simulink model "MotMappedP2"  (R2022a)
settings: Solver=VariableStepAuto  StartTime=0.0  StopTime=inf  RelTol=1e-3  EnableMultiTasking=on
model workspace (MAT data in the model file):
  EV_current = Simulink.Parameter
  EV_current.Value = 200
  EV_current.DataType = 'double'
  EV_current.Complexity = 'real'
  EV_current.Dimensions = [1 1]
  EV_motion = Simulink.Parameter
  EV_motion.Value = [20 4 0.8]
  EV_motion.DataType = 'double'
  EV_motion.Complexity = 'real'
  EV_motion.Dimensions = [1 3]
  EV_sf = Simulink.Parameter
  EV_sf.Value = 2000
  EV_sf.DataType = 'double'
  EV_sf.Complexity = 'real'
  EV_sf.Dimensions = [1 1]
  Fs = Simulink.Parameter
  Fs.Value = 0
  Fs.DataType = 'double'
  Fs.Complexity = 'real'
  Fs.Dimensions = [1 1]
  Fv = Simulink.Parameter
  Fv.Value = 0.0025
  Fv.DataType = 'double'
  Fv.Complexity = 'real'
  Fv.Dimensions = [1 1]
  Jcomp = Simulink.Parameter
  Jcomp.Value = 0.0227
  Jcomp.DataType = 'double'
  Jcomp.Complexity = 'real'
  Jcomp.Dimensions = [1 1]
  Ki = Simulink.Parameter
  Ki.Value = 251.3274
  Ki.DataType = 'double'
  Ki.Complexity = 'real'
  Ki.Dimensions = [1 1]
  Kisa = Simulink.Parameter
  Kisa.Value = 346.6583
  Kisa.DataType = 'double'
  Kisa.Complexity = 'real'
  Kisa.Dimensions = [1 1]
  Kp_d = Simulink.Parameter
  Kp_d.Value = 0.47149
  Kp_d.DataType = 'double'
  Kp_d.Complexity = 'real'
  Kp_d.Dimensions = [1 1]
  Kp_q = Simulink.Parameter
  Kp_q.Value = 0.52125
  Kp_q.DataType = 'double'
  Kp_q.Complexity = 'real'
  Kp_q.Dimensions = [1 1]
  Ksa = Simulink.Parameter
  Ksa.Value = 85.4316
  Ksa.DataType = 'double'
  Ksa.Complexity = 'real'
  Ksa.Dimensions = [1 1]
  Ksf = Simulink.Parameter
  Ksf.Value = 1996.2651
  Ksf.DataType = 'double'
  Ksf.Complexity = 'real'
  Ksf.Dimensions = [1 1]
  Ld = Simulink.Parameter
  Ld.Value = 0.0003752
  Ld.DataType = 'double'
  Ld.Complexity = 'real'
  Ld.Dimensions = [1 1]
  Ldq = Simulink.Parameter
  Ldq.Value = [0.0003752 0.0004148]
  Ldq.DataType = 'double'
  Ldq.Complexity = 'real'
  Ldq.Dimensions = [1 2]
  Lq = Simulink.Parameter
  Lq.Value = 0.0004148
  Lq.DataType = 'double'
  Lq.Complexity = 'real'
  Lq.Dimensions = [1 1]
  Mechanical = Simulink.Parameter
  Mechanical.Value = [0.0227 0.0025 0]
  Mechanical.DataType = 'double'
  Mechanical.Complexity = 'real'
  Mechanical.Dimensions = [1 3]
  P = Simulink.Parameter
  P.Value = 4
  P.DataType = 'double'
  P.Complexity = 'real'
  P.Dimensions = [1 1]
  PolePairs = Simulink.Parameter
  PolePairs.Value = 4
  PolePairs.DataType = 'double'
  PolePairs.Complexity = 'real'
  PolePairs.Dimensions = [1 1]
  Rs = Simulink.Parameter
  Rs.Value = 0.2
  Rs.DataType = 'double'
  Rs.Complexity = 'real'
  Rs.Dimensions = [1 1]
  T_eff_bp = Simulink.Parameter
  T_eff_bp.Value = [0 20 40 60 80 100 120 140 160 180 200]
  T_eff_bp.DataType = 'double'
  T_eff_bp.Complexity = 'real'
  T_eff_bp.Dimensions = [1 11]
  T_max = Simulink.Parameter
  T_max.Value = 120
  T_max.DataType = 'double'
  T_max.Complexity = 'real'
  T_max.Dimensions = [1 1]
  T_mtpa = Simulink.Parameter
  T_mtpa.Value = [0 13.3131834767 26.6278836885 39.9456159322 53.2678926341 66.5962219318 79.9321062746 93.277041051 106.632513247 120.000000141]
  T_mtpa.DataType = 'double'
  T_mtpa.Complexity = 'real'
  T_mtpa.Dimensions = [1 10]
  Tc = Simulink.Parameter
  Tc.Value = 0.02
  Tc.DataType = 'double'
  Tc.Complexity = 'real'
  Tc.Dimensions = [1 1]
  Temp_eff_bp = Simulink.Parameter
  Temp_eff_bp.Value = [233.15 293.15 373.15]
  Temp_eff_bp.DataType = 'double'
  Temp_eff_bp.Complexity = 'real'
  Temp_eff_bp.Dimensions = [1 3]
  ba = Simulink.Parameter
  ba.Value = 3.4029
  ba.DataType = 'double'
  ba.Complexity = 'real'
  ba.Dimensions = [1 1]
  efficiency_table = Simulink.Parameter
  efficiency_table.Value = [52  78  80  82  82  80  78  78  76  74  70; 52  78  80  82  82  80  78  78  76  74  70; 52  78  84  86  86  86  86  84  84  82  82; 52  80  86  86  88  88  88  86  86  84  84; 52  80  86  88  88  88  88  88  86  86  86; 52  80  86  88  90  90  90  90  88  88  88; 52  82  88  90  91  91  92  92  92  91  91; 52  82  88  91  91  92  93  93  93  93  93; 52  84  90  92  92  93  93  93  93  93  93; 62  86  91  93  93  93  93  93  93  93  93; 66  86  91  93  93  93  93  93  93  93  93; 70  86  92  93  93  93  93  93  93  93  93; 70  86  92  93  93  93  93  93  93  93  93; 72  86  91  93  93  93  93  93  93  93  93]
  efficiency_table.DataType = 'double'
  efficiency_table.Complexity = 'real'
  efficiency_table.Dimensions = [14 11]
  efficiency_table_3d = Simulink.Parameter
  efficiency_table_3d.Value = reshape([92 92 92 92 92 92 92 92 92 92 92 92 92 92 92 92 92 92 92 92 92 92 92 92 92 92 92 92 92 92 92 92 92 92 92 92 92 92 92 92 92 92 92 92 92 92 92 92 92 92 92 92 92 92 92 92 92 92 92 92 92 92 92 92 92 92 92 92 92 92 92 92 92 92 92 92 92 92 92 92 92 92 92 92 92 92 92 92 92 92 92 92 92 92 92 92 92 92 92 92 92 92 92 92 92 92 92 92 92 92 92 92 92 92 92 92 92 92 92 92 92 92 92 92 92 92 92 92 92 92 92 92 92 92 92 92 92 92 92 92 92 92 92 92 92 92 92 92 92 92 92 92 92 92 95 95 95 95 95 95 95 95 95 95 95 95 95 95 95 95 95 95 95 95 95 95 95 95 95 95 95 95 95 95 95 95 95 95 95 95 95 95 95 95 95 95 95 95 95 95 95 95 95 95 95 95 95 95 95 95 95 95 95 95 95 95 95 95 95 95 95 95 95 95 95 95 95 95 95 95 95 95 95 95 95 95 95 95 95 95 95 95 95 95 95 95 95 95 95 95 95 95 95 95 95 95 95 95 95 95 95 95 95 95 95 95 95 95 95 95 95 95 95 95 95 95 95 95 95 95 95 95 95 95 95 95 95 95 95 95 95 95 95 95 95 95 95 95 95 95 95 95 95 95 95 95 95 95 93 93 93 93 93 93 93 93 93 93 93 93 93 93 93 93 93 93 93 93 93 93 93 93 93 93 93 93 93 93 93 93 93 93 93 93 93 93 93 93 93 93 93 93 93 93 93 93 93 93 93 93 93 93 93 93 93 93 93 93 93 93 93 93 93 93 93 93 93 93 93 93 93 93 93 93 93 93 93 93 93 93 93 93 93 93 93 93 93 93 93 93 93 93 93 93 93 93 93 93 93 93 93 93 93 93 93 93 93 93 93 93 93 93 93 93 93 93 93 93 93 93 93 93 93 93 93 93 93 93 93 93 93 93 93 93 93 93 93 93 93 93 93 93 93 93 93 93 93 93 93 93 93 93], [14 11 3])
  efficiency_table_3d.DataType = 'double'
  efficiency_table_3d.Complexity = 'real'
  efficiency_table_3d.Dimensions = [14 11 3]
  id_mtpa = Simulink.Parameter
  id_mtpa.Value = [0 -0.114523352646 -0.457989076459 -1.03008464374 -1.83029075221 -2.85788367342 -4.11193850568 -5.59133329791 -7.29475400168 -9.22070020138]
  id_mtpa.DataType = 'double'
  id_mtpa.Complexity = 'real'
  id_mtpa.Dimensions = [1 10]
  idq0 = Simulink.Parameter
  idq0.Value = [0 0]
  idq0.DataType = 'double'
  idq0.Complexity = 'real'
  idq0.Dimensions = [1 2]
  idq_limits = Simulink.Parameter
  idq_limits.Value = [-9.220699542 166.993501392 167.247872355]
  idq_limits.DataType = 'double'
  idq_limits.Complexity = 'real'
  idq_limits.Dimensions = [1 3]
  iq_mtpa = Simulink.Parameter
  iq_mtpa.Value = [0 18.5827440345 37.1633719111 55.7397734896 74.3098506185 92.871523015 111.422734008 129.961456105 148.485696337 166.993501356]
  iq_mtpa.DataType = 'double'
  iq_mtpa.Complexity = 'real'
  iq_mtpa.Dimensions = [1 10]
  lambda_pm = Simulink.Parameter
  lambda_pm.Value = 0.1194
  lambda_pm.DataType = 'double'
  lambda_pm.Complexity = 'real'
  lambda_pm.Dimensions = [1 1]
  losses_table = Simulink.Parameter
  losses_table.Value = [0 0 0 0 0 0 0 0 0 0 0 0 ... (154 elements, 14x11)]
  losses_table.DataType = 'double'
  losses_table.Complexity = 'real'
  losses_table.Dimensions = [14 11]
  losses_table_3d = Simulink.Parameter
  losses_table_3d.Value = reshape([2 2 2 2 2 2 2 2 2 2 2 2 2 2 2 2 2 2 2 2 2 2 2 2 2 2 2 2 2 2 2 2 2 2 2 2 2 2 2 2 2 2 2 2 2 2 2 2 2 2 2 2 2 2 2 2 2 2 2 2 2 2 2 2 2 2 2 2 2 2 2 2 2 2 2 2 2 2 2 2 2 2 2 2 2 2 2 2 2 2 2 2 2 2 2 2 2 2 2 2 2 2 2 2 2 2 2 2 2 2 2 2 2 2 2 2 2 2 2 2 2 2 2 2 2 2 2 2 2 2 2 2 2 2 2 2 2 2 2 2 2 2 2 2 2 2 2 2 2 2 2 2 2 2 1.5 1.5 1.5 1.5 1.5 1.5 1.5 1.5 1.5 1.5 1.5 1.5 1.5 1.5 1.5 1.5 1.5 1.5 1.5 1.5 1.5 1.5 1.5 1.5 1.5 1.5 1.5 1.5 1.5 1.5 1.5 1.5 1.5 1.5 1.5 1.5 1.5 1.5 1.5 1.5 1.5 1.5 1.5 1.5 1.5 1.5 1.5 1.5 1.5 1.5 1.5 1.5 1.5 1.5 1.5 1.5 1.5 1.5 1.5 1.5 1.5 1.5 1.5 1.5 1.5 1.5 1.5 1.5 1.5 1.5 1.5 1.5 1.5 1.5 1.5 1.5 1.5 1.5 1.5 1.5 1.5 1.5 1.5 1.5 1.5 1.5 1.5 1.5 1.5 1.5 1.5 1.5 1.5 1.5 1.5 1.5 1.5 1.5 1.5 1.5 1.5 1.5 1.5 1.5 1.5 1.5 1.5 1.5 1.5 1.5 1.5 1.5 1.5 1.5 1.5 1.5 1.5 1.5 1.5 1.5 1.5 1.5 1.5 1.5 1.5 1.5 1.5 1.5 1.5 1.5 1.5 1.5 1.5 1.5 1.5 1.5 1.5 1.5 1.5 1.5 1.5 1.5 1.5 1.5 1.5 1.5 1.5 1.5 1.5 1.5 1.5 1.5 1.5 1.5 1.9 1.9 1.9 1.9 1.9 1.9 1.9 1.9 1.9 1.9 1.9 1.9 1.9 1.9 1.9 1.9 1.9 1.9 1.9 1.9 1.9 1.9 1.9 1.9 1.9 1.9 1.9 1.9 1.9 1.9 1.9 1.9 1.9 1.9 1.9 1.9 1.9 1.9 1.9 1.9 1.9 1.9 1.9 1.9 1.9 1.9 1.9 1.9 1.9 1.9 1.9 1.9 1.9 1.9 1.9 1.9 1.9 1.9 1.9 1.9 1.9 1.9 1.9 1.9 1.9 1.9 1.9 1.9 1.9 1.9 1.9 1.9 1.9 1.9 1.9 1.9 1.9 1.9 1.9 1.9 1.9 1.9 1.9 1.9 1.9 1.9 1.9 1.9 1.9 1.9 1.9 1.9 1.9 1.9 1.9 1.9 1.9 1.9 1.9 1.9 1.9 1.9 1.9 1.9 1.9 1.9 1.9 1.9 1.9 1.9 1.9 1.9 1.9 1.9 1.9 1.9 1.9 1.9 1.9 1.9 1.9 1.9 1.9 1.9 1.9 1.9 1.9 1.9 1.9 1.9 1.9 1.9 1.9 1.9 1.9 1.9 1.9 1.9 1.9 1.9 1.9 1.9 1.9 1.9 1.9 1.9 1.9 1.9 1.9 1.9 1.9 1.9 1.9 1.9], [14 11 3])
  losses_table_3d.DataType = 'double'
  losses_table_3d.Complexity = 'real'
  losses_table_3d.Dimensions = [14 11 3]
  mechanical = Simulink.Parameter
  mechanical.Value = [0.0227 0.0025 0]
  mechanical.DataType = 'double'
  mechanical.Complexity = 'real'
  mechanical.Dimensions = [1 3]
  omega_init = Simulink.Parameter
  omega_init.Value = 0
  omega_init.DataType = 'double'
  omega_init.Complexity = 'real'
  omega_init.Dimensions = [1 1]
  power_max = Simulink.Parameter
  power_max.Value = 30000
  power_max.DataType = 'double'
  power_max.Complexity = 'real'
  power_max.Dimensions = [1 1]
  theta_init = Simulink.Parameter
  theta_init.Value = 0
  theta_init.DataType = 'double'
  theta_init.Complexity = 'real'
  theta_init.Dimensions = [1 1]
  torque_max = Simulink.Parameter
  torque_max.Value = 200
  torque_max.DataType = 'double'
  torque_max.Complexity = 'real'
  torque_max.Dimensions = [1 1]
  w_eff_bp = Simulink.Parameter
  w_eff_bp.Value = [0 52.3598775598 104.71975512 149.999649207 157.079632679 209.439510239 261.799387799 314.159265359 366.519142919 418.879020479 471.238898038 523.598775598 575.958653158 628.318530718]
  w_eff_bp.DataType = 'double'
  w_eff_bp.Complexity = 'real'
  w_eff_bp.Dimensions = [1 14]
libraries: autolibmappedmotor x1
settings Model: DataDictionary=MotMappedP2.sldd  ModifiedByFormat=The MathWorks, Inc.  PauseTimes=10  Creator=The MathWorks, Inc.  LastModifiedBy=The MathWorks, Inc.
settings SolverCC: AlgebraicLoopSolver=TrustRegion  AutoInsertRateTranBlk=on  DecoupledContinuousIntegration=on  MaxZcPerStep=1
settings DataIOCC: DSMLogging=off  ReturnWorkspaceOutputs=off
settings DebuggingCC: UnconnectedInputMsg=warning  UnconnectedOutputMsg=warning  UnconnectedLineMsg=warning  PregeneratedLibrarySubsystemCodeDiagnostic=none  SFMachineParentedDataDiag=warning  ArithmeticOperatorsInVariantConditions=warning
settings ModelReferenceCC: PropagateSignalLabelsOutOfModel=off
settings SFSimCC: SimUseLocalCustomCode=off  CustomCodeUndefinedFunction=UseInterfaceOnly
settings RTWCC: RTWUseLocalCustomCode=off  DLArmComputeVersion=19.05
settings CodeAppCC: StateflowObjectComments=on
settings GRTTargetCC: TargetLangStandard=C89/C90 (ANSI)
settings ConfigComp: CovMetricSettings=dsw  CovSaveCumulativeToWorkspaceVar=on  CovSaveSingleToWorkspaceVar=on  CovExternalEMLEnable=off
settings SimscapeCC: SimscapeNormalizeSystem=off

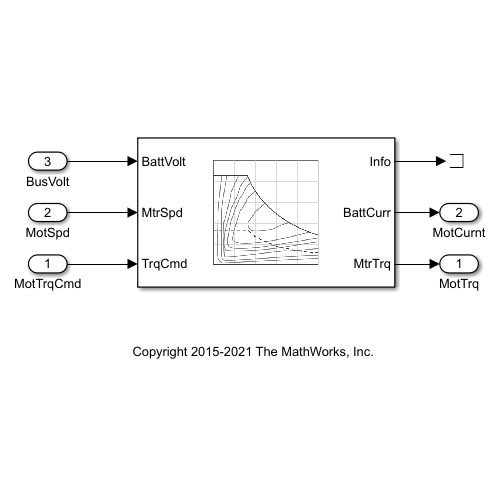
[thumbnail: Simulink's stored preview of the top-level diagram]
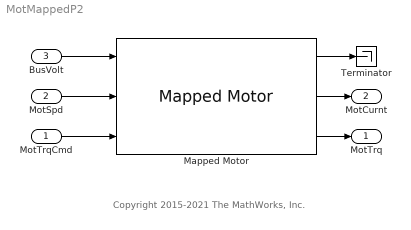
== system MotMappedP2 ==
  note: Copyright 2015-2021 The MathWorks, Inc.
  MotTrqCmd : Inport
  MotSpd : Inport  Port=2
  BusVolt : Inport  Port=3
  Mapped Motor : autolibmappedmotor/Mapped Motor  port_config=Speed  param_by=Maximum torque and power  w_t=[ 0 375 750 800 ]  T_t=[0.09 0.08 0.07 0]  torque_max=torque_max  power_max=power_max  Tc=Tc  param_loss=Tabulated efficiency data  eff=100  w_eff=375  T_eff=0.08  Piron=0  Pbase=0  w_eff_bp=w_eff_bp  T_eff_bp=T_eff_bp  Temp_eff_bp=Temp_eff_bp  losses_table=losses_table  losses_table_3d=losses_table_3d  efficiency_table=efficiency_table  efficiency_table_3d=efficiency_table_3d  J=5e-6  b=1e-5  omega_o=0  T_t_extended=[0 0.07 0.08 0.09 0.08 0.07 0]  w_t_extended=[-800 -750 -375 0 375 750 800]  KLossIron=0  KLossCopper=0  x_w_eff_vec=[-628.318530717959 -575.958653158129 -523.598775598299 -471.238898038469 -418.879020478639 -366.519142918809 -314.159265358979 -261.799387799149 -209.43951023932 -157.07963267949 -149.999649206931 -104.71975511966 -52.3598775598299 0 52.3598775598299 104.71975511966 149.999649206931 157.07963267949 209.43951023932 261.799387799149 314.159265358979 366.519142918809 418.879020478639 471.238898038469 523.598775598299 575.958653158129 628.318530717959]  x_T_eff_vec=[-200 -180 -160 -140 -120 -100 -80 -60 -40 -20 0 20 40 60 80 100 120 140 160 180 200]  x_tmp_eff_vec=[233.15 293.15 373.15]  x_losses_mat=[9458.558526937 8512.7026742433 7566.8468215496 6620.9909688559 5675.1351161622 4729.2792634685 3783.4234107748 2837.5675580811 2485.6557259172 2045.68823954684 0 1759.29188601028 2261.94671058465 2638.93782901542 3518.58377202057 4398.22971502571 5277.87565803085 6157.52160103599 7037.16754404113 7916.81348704627 8796.45943005141;8670.34531635892 7803.31078472303 6936.27625308713 6069.24172145124 5202.20718981535 4335.17265817946 3468.13812654357 2601.10359490768 2003.3344457674 1875.21421958461 0 1612.68422884276 1843.06769010601 2419.02634326414 3225.36845768552 4031.7105721069 4838.05268652828 5644.39480094966 6450.73691537104 7257.07902979242 8063.4211442138;7882.13210578084 7093.91889520275 6305.70568462467 5517.49247404659 4729.2792634685 3941.06605289042 3152.85284231233 2364.63963173425 1821.21313251582 1704.74019962237 0 1466.07657167524 1675.51608191456 2199.11485751285 2932.15314335047 3665.19142918809 4398.22971502571 5131.26800086333 5864.30628670094 6597.34457253856 7330.38285837618;7093.91889520275 6384.52700568248 5675.1351161622 4965.74322664193 4256.35133712165 3546.95944760138 2837.5675580811 2128.17566856083 1864.2417944379 1534.26617966013 0 1319.46891450771 1696.46003293849 1979.20337176157 2638.93782901542 3298.67228626928 3958.40674352314 4618.14120077699 5277.87565803085 5937.61011528471 6597.34457253856;6305.70568462467 5675.1351161622 5044.56454769974 4413.99397923727 3783.4234107748 3152.85284231233 2522.28227384987 1891.7117053874 1657.10381727813 1363.7921596979 0 1172.86125734019 1507.9644737231 1759.29188601028 2345.72251468038 2932.15314335047 3518.58377202057 4105.01440069066 4691.44502936075 5277.87565803085 5864.30628670094;5517.49247404658 4965.74322664193 4413.99397923727 3862.24473183261 3310.49548442795 2758.74623702329 2549.69838552215 1912.27378914161 1628.97396852804 1396.26340159546 0 1172.86125734019 1466.07657167524 1759.29188601028 2345.72251468038 2565.63400043166 3078.76080051799 3591.88760060433 4105.01440069066 4618.14120077699 5131.26800086332;4729.2792634685 4256.35133712165 3783.4234107748 3310.49548442795 2837.5675580811 2731.81969877373 2485.6557259172 1864.2417944379 1713.59599286716 1379.23579913698 0 1130.97335529233 1507.9644737231 1696.46003293849 2261.94671058465 2513.27412287183 2638.93782901542 3078.760800518 3518.58377202057 3958.40674352314 4398.22971502571;5178.44942899416 4660.60448609474 3642.42626503164 3187.12298190269 2731.81969877373 2589.22471449708 2071.37977159766 1745.32925199433 1427.99666072263 1149.36316594749 0 942.477796076938 1256.63706143592 1570.7963267949 1884.95559215388 2356.19449019234 2513.27412287183 2932.15314335047 3351.03216382911 4241.15008234622 4712.38898038469;5711.98664289054 5140.78797860148 4569.58931431243 3257.94793705608 2792.52680319093 2327.10566932577 1861.68453546062 1713.59599286716 1363.7921596979 1047.1975511966 0 837.758040957278 1172.86125734019 1507.9644737231 1675.51608191456 2094.39510239319 2513.27412287183 2932.15314335047 4021.23859659494 4523.8934211693 5026.54824574367;5114.22059886711 4602.7985389804 4091.37647909369 2998.79298751753 2570.39398930074 2141.99499108395 1713.59599286716 1285.19699465037 1022.84411977342 785.398163397448 0 628.318530717959 879.645943005142 1130.97335529233 1507.9644737231 1884.95559215388 2261.94671058465 2638.93782901543 3518.58377202057 3958.40674352314 4398.22971502571;5714.27235074022 5142.8451156662 3906.96760725029 3418.596656344 2454.53971429523 2045.44976191269 1636.35980953016 1465.11285271886 976.741901812573 749.998246034654 0 599.998596827723 839.998035558812 1259.99705333822 1439.99663238654 1799.99579048317 2159.9949485798 2939.99312445584 3359.99214223525 4319.98989715961 4799.98877462179;4597.45266378994 4137.70739741095 3191.45920364677 2792.52680319093 2045.68823954684 1704.74019962237 1363.7921596979 1022.84411977342 797.864800911693 590.726823751927 0 460.766922526503 670.206432765823 879.645943005142 1172.86125734019 1466.07657167524 1759.29188601028 ...(+4852 chars)]  x_losses_mat_3d=cat(3,[2 2 2 2 2 2 2 2 2 2 2 2 2 2 2 2 2 2 2 2 2;2 2 2 2 2 2 2 2 2 2 2 2 2 2 2 2 2 2 2 2 2;2 2 2 2 2 2 2 2 2 2 2 2 2 2 2 2 2 2 2 2 2;2 2 2 2 2 2 2 2 2 2 2 2 2 2 2 2 2 2 2 2 2;2 2 2 2 2 2 2 2 2 2 2 2 2 2 2 2 2 2 2 2 2;2 2 2 2 2 2 2 2 2 2 2 2 2 2 2 2 2 2 2 2 2;2 2 2 2 2 2 2 2 2 2 2 2 2 2 2 2 2 2 2 2 2;2 2 2 2 2 2 2 2 2 2 2 2 2 2 2 2 2 2 2 2 2;2 2 2 2 2 2 2 2 2 2 2 2 2 2 2 2 2 2 2 2 2;2 2 2 2 2 2 2 2 2 2 2 2 2 2 2 2 2 2 2 2 2;2 2 2 2 2 2 2 2 2 2 2 2 2 2 2 2 2 2 2 2 2;2 2 2 2 2 2 2 2 2 2 2 2 2 2 2 2 2 2 2 2 2;2 2 2 2 2 2 2 2 2 2 2 2 2 2 2 2 2 2 2 2 2;2 2 2 2 2 2 2 2 2 2 2 2 2 2 2 2 2 2 2 2 2;2 2 2 2 2 2 2 2 2 2 2 2 2 2 2 2 2 2 2 2 2;2 2 2 2 2 2 2 2 2 2 2 2 2 2 2 2 2 2 2 2 2;2 2 2 2 2 2 2 2 2 2 2 2 2 2 2 2 2 2 2 2 2;2 2 2 2 2 2 2 2 2 2 2 2 2 2 2 2 2 2 2 2 2;2 2 2 2 2 2 2 2 2 2 2 2 2 2 2 2 2 2 2 2 2;2 2 2 2 2 2 2 2 2 2 2 2 2 2 2 2 2 2 2 2 2;2 2 2 2 2 2 2 2 2 2 2 2 2 2 2 2 2 2 2 2 2;2 2 2 2 2 2 2 2 2 2 2 2 2 2 2 2 2 2 2 2 2;2 2 2 2 2 2 2 2 2 2 2 2 2 2 2 2 2 2 2 2 2;2 2 2 2 2 2 2 2 2 2 2 2 2 2 2 2 2 2 2 2 2;2 2 2 2 2 2 2 2 2 2 2 2 2 2 2 2 2 2 2 2 2;2 2 2 2 2 2 2 2 2 2 2 2 2 2 2 2 2 2 2 2 2;2 2 2 2 2 2 2 2 2 2 2 2 2 2 2 2 2 2 2 2 2],[1.5 1.5 1.5 1.5 1.5 1.5 1.5 1.5 1.5 1.5 1.5 1.5 1.5 1.5 1.5 1.5 1.5 1.5 1.5 1.5 1.5;1.5 1.5 1.5 1.5 1.5 1.5 1.5 1.5 1.5 1.5 1.5 1.5 1.5 1.5 1.5 1.5 1.5 1.5 1.5 1.5 1.5;1.5 1.5 1.5 1.5 1.5 1.5 1.5 1.5 1.5 1.5 1.5 1.5 1.5 1.5 1.5 1.5 1.5 1.5 1.5 1.5 1.5;1.5 1.5 1.5 1.5 1.5 1.5 1.5 1.5 1.5 1.5 1.5 1.5 1.5 1.5 1.5 1.5 1.5 1.5 1.5 1.5 1.5;1.5 1.5 1.5 1.5 1.5 1.5 1.5 1.5 1.5 1.5 1.5 1.5 1.5 1.5 1.5 1.5 1.5 1.5 1.5 1.5 1.5;1.5 1.5 1.5 1.5 1.5 1.5 1.5 1.5 1.5 1.5 1.5 1.5 1.5 1.5 1.5 1.5 1.5 1.5 1.5 1.5 1.5;1.5 1.5 1.5 1.5 1.5 1.5 1.5 1.5 1.5 1.5 1.5 1.5 1.5 1.5 1.5 1.5 1.5 1.5 1.5 1.5 1.5;1.5 1.5 1.5 1.5 1.5 1.5 1.5 1.5 1.5 1.5 1.5 1.5 1.5 1.5 1.5 1.5 1.5 1.5 1.5 1.5 1.5;1.5 1.5 1.5 1.5 1.5 1.5 1.5 1.5 1.5 1.5 1.5 1.5 1.5 1.5 1.5 1.5 1.5 1.5 1.5 1.5 1.5;1.5 1.5 1.5 1.5 1.5 1.5 1.5 1.5 1.5 1.5 1.5 1.5 1.5 1.5 1.5 1.5 1.5 1.5 1.5 1.5 1.5;1.5 1.5 1.5 1.5 1.5 1.5 1.5 1.5 1.5 1.5 1.5 1.5 1.5 1.5 1.5 1.5 1.5 1.5 1.5 1.5 1.5;1.5 1.5 1.5 1.5 1.5 1.5 1.5 1.5 1.5 1.5 1.5 1.5 1.5 1.5 1.5 1.5 1.5 1.5 1.5 1.5 1.5;1.5 1.5 1.5 1.5 1.5 1.5 1.5 1.5 1.5 1.5 1.5 1.5 1.5 1.5 1.5 1.5 1.5 1.5 1.5 1.5 1.5;1.5 1.5 1.5 1.5 1.5 1.5 1.5 1.5 1.5 1.5 1.5 1.5 1.5 1.5 1.5 1.5 1.5 1.5 1.5 1.5 1.5;1.5 1.5 1.5 1.5 1.5 1.5 1.5 1.5 1.5 1.5 1.5 1.5 1.5 1.5 1.5 1.5 1.5 1.5 1.5 1.5 1.5;1.5 1.5 1.5 1.5 1.5 1.5 1.5 1.5 1.5 1.5 1.5 1.5 1.5 1.5 1.5 1.5 1.5 1.5 1.5 1.5 1.5;1.5 1.5 1.5 1.5 1.5 1.5 1.5 1.5 1.5 1.5 1.5 1.5 1.5 1.5 1.5 1.5 1.5 1.5 1.5 1.5 1.5;1.5 1.5 1.5 1.5 1.5 1.5 1.5 1.5 1.5 1.5 1.5 1.5 1.5 1.5 1.5 1.5 1.5 1.5 1.5 1.5 1.5;1.5 1.5 1.5 1.5 1.5 1.5 1.5 1.5 1.5 1.5 1.5 1.5 1.5 1.5 1.5 1.5 1.5 1.5 1.5 1.5 1.5;1.5 1.5 1.5 1.5 1.5 1.5 1.5 1.5 1.5 1.5 1.5 1.5 1.5 1.5 1.5 1.5 1.5 1.5 1.5 1.5 1.5;1.5 1.5 1.5 1.5 1.5 1.5 1.5 1.5 1.5 1.5 1.5 1.5 1.5 1.5 1.5 1.5 1.5 1.5 1.5 1.5 1.5;1.5 1.5 1.5 1.5 1.5 1.5 1.5 1.5 1.5 1.5 1.5 1.5 1.5 1.5 1.5 1.5 1.5 1.5 1.5 1.5 1.5;1.5 1.5 1.5 1.5 1.5 1.5 1.5 1.5 1.5 1.5 1.5 1.5 1.5 1.5 1.5 1.5 1.5 1.5 1.5 1.5 1.5;1.5 1.5 1.5 1.5 1.5 1.5 1.5 1.5 1.5 1.5 1.5 1.5 1.5 1.5 1.5 1.5 1.5 1.5 1.5 1.5 1.5;1.5 1.5 1.5 1.5 1.5 1.5 1.5 1.5 1.5 1.5 1.5 1.5 1.5 1.5 1.5 1.5 1.5 1.5 1.5 1.5 1.5;1.5 1.5 1.5 1.5 1.5 1.5 1.5 1.5 1.5 1.5 1.5 1.5 1.5 1.5 1.5 1.5 1.5 1.5 1.5 1.5 1.5;1.5 1.5 1.5 1.5 1.5 1.5 1.5 1.5 1.5 1.5 1.5 1.5 1.5 1.5 1.5 1.5 1.5 1.5 1.5 1.5 1.5],[1.9 1.9 1.9 1.9 1.9 1.9 1.9 1.9 1.9 1.9 1.9 1.9 1.9 1.9 1.9 1.9 1.9 1.9 1.9 1.9 1.9;1.9 1.9 1.9 1.9 1.9 1.9 1.9 1.9 1.9 1.9 1.9 1.9 1.9 1.9 1.9 1.9 1.9 1.9 1.9 1.9 1.9;1.9 1.9 1.9 1.9 1.9 1.9 1.9 1.9 1.9 1.9 1.9 1.9 1.9 1.9 1.9 1.9 1.9 1.9 1.9 1.9 1.9;1.9 1.9 1.9 1.9 1.9 1.9 1.9 1.9 1.9 1.9 1.9 1.9 1.9 1.9 1.9 1.9 1.9 1.9 1.9 1.9 1.9;1.9 1.9 1.9 1.9 1.9 1.9 1.9 1.9 1.9 1.9 1.9 1.9 1.9 1.9 1.9 1.9 1.9 1.9 1.9 1.9 1.9;1.9 1.9 1.9 1.9 1.9 1.9 1.9 1.9 1.9 1.9 1.9 1.9 1.9 1.9 1.9 1.9 1.9 1.9 1.9 1.9 1.9;1.9 1.9 1.9 1.9 1.9 1.9 1.9 1.9 1.9 1.9 1.9 1.9 1.9 1.9 1.9 1.9 1.9 1.9 1.9 1.9 1.9 ...(+1680 chars)])  CalLossMapData={'BaseCageProjectFileName','';'BaseMbcProjectFileName','';'TaskName','Calibrate Motor Loss Map';'ChildTasks',{{'DataName','';'TaskName','Import Loss Data'},{'TaskName','Generate Response Models'},{'TaskName','Generate Calibration'},{'TaskName','Update Block Parameters'}}}  CalLossWithTempMapData={}  aMode=aMode  RefBlkName='autolibmappedmotor/Mapped Motor'
      settings: SourceProductBaseCode=PW,DR,MT,VE
  Terminator : Terminator
  MotTrq : Outport  VectorParamsAs1DForOutWhenUnconnected=off
  MotCurnt : Outport  Port=2  VectorParamsAs1DForOutWhenUnconnected=off
  wires:
  MotTrqCmd/1 -> Mapped Motor/3
  BusVolt/1 -> Mapped Motor/1
  MotSpd/1 -> Mapped Motor/2
  Mapped Motor/3 -> MotTrq/1
  Mapped Motor/2 -> MotCurnt/1
  Mapped Motor/1 -> Terminator/1
